simulink model "distributed_project_square"  (R2025b)
settings: Solver=VariableStepAuto  StartTime=0.0  StopTime=10  RelTol=1e-3  AbsTol=1e-3  EnableMultiTasking=on
model workspace (MAT data in the model file):
  t_now = 10
  v = 1
values from neighbouring files (symbols this model uses):
  m = 20    [FirstRegression.m]
  msg_init =     [distributed_project_adjusted.mat]
  N = min([length(e1), length(e2), length(e3), N_max])    [10_runs_result_for_odometer.m]    (also in cc.m = min(length(e1), length(e2)); distributed_project_adjusted.mat = 100; distributed_stats.m = min([length(e1),length(e2),length(e3)]); ten_runs_result_for_odometer.m)
  r = 0.05    [distributed_project.mat]    (also in distributed_project_adjusted.mat)
undefined symbols (not defined in the file or in its folder): fractalcoef, X, Y, Z
libraries: nesl_utility x69, sm_lib x50, simulink x20, matrix_library x20, mspfiltlib x4, sensorgpslib x4, mspsensorlib x4
(part 1 of 5)
settings Model: Creator=root  LastModifiedBy=root
settings SolverCC: AutoScaleAbsTol=off  AlgebraicLoopSolver=TrustRegion  MaxZcPerStep=1.0
settings DataIOCC: LimitDataPoints=on  MaxDataPoints=10000
settings OptimizationCC: ReuseModelBlockBuffer=off  LifeSpan=inf
settings DebuggingCC: UnconnectedInputMsg=warning  UnconnectedOutputMsg=warning  UnconnectedLineMsg=warning  AllowSymbolicDim=off  SubsystemReferenceDiagnosticForUnitTest=warning  SFUnexpectedBacktrackingDiag=warning  SFNoUnconditionalDefaultTransitionDiag=warning  SFExecutionAtInitializationDiag=none  UnderSpecifiedDimensionMsg=warning  ArithmeticOperatorsInVariantConditions=warning
settings ModelReferenceCC: EnableRefExpFcnMdlSchedulingChecks=on
settings SFSimCC: SimUseLocalCustomCode=off  CustomCodeUndefinedFunction=UseInterfaceOnly
settings RTWCC: RTWUseLocalCustomCode=off  GPUComputeCapability=3.5  DLArmComputeVersion=19.05
settings CodeAppCC: StateflowObjectComments=on
settings GRTTargetCC: TargetLangStandard=C89/C90 (ANSI)
settings ConfigComp: CovMetricSettings=dw  CovSaveCumulativeToWorkspaceVar=on  CovSaveSingleToWorkspaceVar=on  CovExternalEMLEnable=off  CovSFcnEnable=off
settings SimscapeCC: SimscapeLogType=all  SimscapeLogSimulationStatistics=on  SimscapeLogDataHistory=10000.0

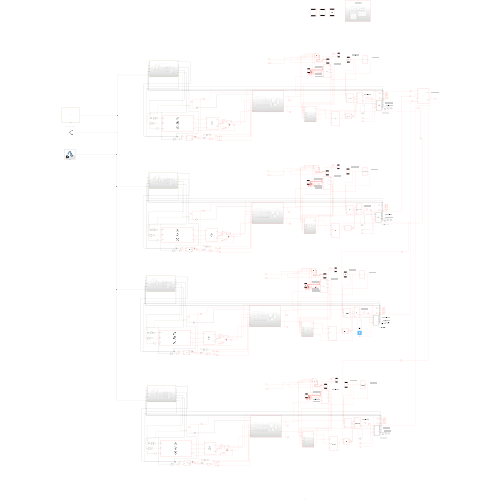
[thumbnail: Simulink's stored preview of the top-level diagram]
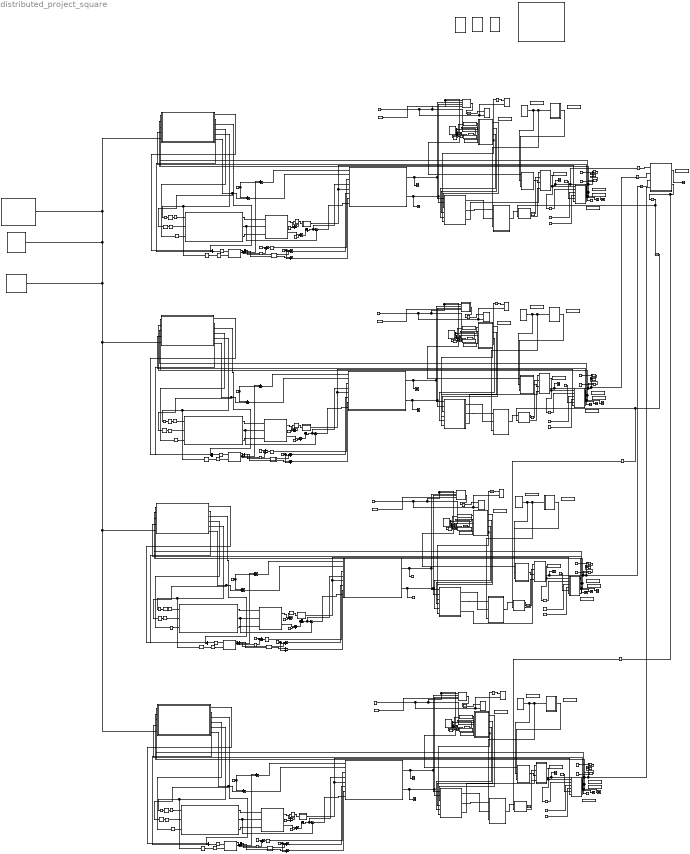
== system distributed_project_square ==
  AHRS{,1..3} (4 alike) : mspfiltlib/AHRS  DispRefFrame=NED  DecimationFactor=1  InitialProcessNoise=ahrsfilter.defaultProcessNoise  OrientationFormat=quaternion  SimulateUsing=Interpreted execution  AccelerometerNoise=0.0001924722  GyroscopeNoise=9.1385e-5  MagnetometerNoise=0.1  GyroscopeDriftNoise=3.0462e-13  LinearAccelerationNoise=0.0096236100000000012  MagneticDisturbanceNoise=0.5  LinearAccelerationDecayFactor=0.5  MagneticDisturbanceDecayFactor=0.5  ExpectedMagneticFieldStrength=50
  Add{1..28} (28 alike) : Sum
  Band-Limited White Noise{,1..19} (20 alike) : simulink/Sources/Band-Limited White Noise  Cov=[0.1]  Ts=0.01  seed=[23341]
  Bus Selector{,1..3} (4 alike) : BusSelector  OutputSignals=ID,x,P,t
  Constant : Constant  Value=2  OutDataTypeStr=int32  SampleTime=0.01
  Constant1 : Constant  OutDataTypeStr=int32  SampleTime=0.01
  Constant{4,7,10..11} (4 alike) : Constant  Value=0.8  SampleTime=0.01
  Constant2 : Constant  Value=3  OutDataTypeStr=int32  SampleTime=0.01
  Constant{3,6,8..9} (4 alike) : Constant  Value=0.0  SampleTime=0.01
  Constant5 : Constant  Value=4  OutDataTypeStr=int32  SampleTime=0.01
  Data Store Memory : DataStoreMemory  DataStoreName=msg_in  WriteAfterWriteMsg=warning  InitialValue=msg_init  ShowAdditionalParam=off  OutDataTypeStr=Bus: msgBus  Dimensions=MAX_AGENTS
  Data Store Memory1 : DataStoreMemory  DataStoreName=N  WriteAfterWriteMsg=warning  InitialValue=1  ShowAdditionalParam=off  OutDataTypeStr=double  Dimensions=MAX_AGENTS
  Data Store Memory2 : DataStoreMemory  DataStoreName=N_final  WriteAfterWriteMsg=warning  InitialValue=MAX_AGENTS  ShowAdditionalParam=off
  Data Store Read{,2,4,6} (4 alike) : DataStoreRead  DataStoreName=msg_in  SampleTime=0.01  DataStoreElements=msg_in  IndexOptions=Index vector (dialog)  Indices=1  OutputSizes=1
  Data Store Read{1,3,5,7} (4 alike) : DataStoreRead  DataStoreName=N_final  SampleTime=0.01  IndexOptions=Index vector (dialog)  Indices=1  OutputSizes=1
  Data Store Write{,2,4,6} (4 alike) : DataStoreWrite  DataStoreName=msg_in  SampleTime=0.01  DataStoreElements=msg_in  EnableIndexing=on  IndexOptions=Index vector (port)  Indices=1  OutputSizes=1
  Data Store Write{1,3,5,7} (4 alike) : DataStoreWrite  DataStoreName=N  SampleTime=0.01  EnableIndexing=on  IndexOptions=Index vector (port)  Indices=1  OutputSizes=1
  Demux{1..8} (8 alike) : Demux  Outputs=3
  Derivative{,1..11} (12 alike) : Derivative
  Digital Clock{,1..7} (8 alike) : DigitalClock  SampleTime=0.01
  Display{,1..40} (41 alike) : DisplayBlock  LabelPosition=Hide  Transparency=1  GridColor=[0.502, 0.502, 0.502]
  GPS{,1..3} (4 alike) : sensorgpslib/GPS  DispRefFrame=NED  PositionInputFormat=Local  ReferenceLocation=[ 0, 0, 0 ]  HorizontalPositionAccuracy=1.6  VerticalPositionAccuracy=3  VelocityAccuracy=0.1  DecayFactor=0.999  SeedDouble=67  SimulateUsing=Interpreted execution
      settings: LibrarySourceBlock=mspsensorlib/GPS
  IMU{,1..3} (4 alike) : mspsensorlib/IMU  DispRefFrame=NED  TemperaturePort=off  Temperature=25  MagneticFieldPort=off  MagneticFieldNED=[ 27.5550, -2.4169, -16.0849 ]  MagneticFieldENU=[ -2.4169, 27.5550, 16.0849 ]  SeedDouble=67  SimulateUsing=Interpreted execution  AccelParamsMeasurementRange=Inf  AccelParamsResolution=0  AccelParamsConstantBias=[ 0, 0, 0 ]  AccelParamsAxesMisalignment=[ 100, 0, 0; 0, 100, 0; 0, 0, 100 ]  AccelParamsNoiseDensity=[ 0, 0, 0 ]  AccelParamsBiasInstability=[ 0, 0, 0 ]  AccelParamsBiasInstabilityNumerator=fractalcoef().Numerator  AccelParamsBiasInstabilityDenominator=fractalcoef().Denominator  AccelParamsRandomWalk=[ 0, 0, 0 ]  AccelParamsNoiseType=double-sided  AccelParamsTemperatureBias=[ 0, 0, 0 ]  AccelParamsTemperatureScaleFactor=[ 0, 0, 0 ]  GyroParamsMeasurementRange=Inf  GyroParamsResolution=0  GyroParamsConstantBias=[ 0, 0, 0 ]  GyroParamsAxesMisalignment=[ 100, 0, 0; 0, 100, 0; 0, 0, 100 ]  GyroParamsAccelerationBias=[ 0, 0, 0 ]  GyroParamsNoiseDensity=[ 0, 0, 0 ]  GyroParamsBiasInstability=[ 0, 0, 0 ]  GyroParamsBiasInstabilityNumerator=fractalcoef().Numerator  GyroParamsBiasInstabilityDenominator=fractalcoef().Denominator  GyroParamsRandomWalk=[ 0, 0, 0 ]  GyroParamsNoiseType=double-sided  GyroParamsTemperatureBias=[ 0, 0, 0 ]  GyroParamsTemperatureScaleFactor=[ 0, 0, 0 ]  MagParamsMeasurementRange=Inf  MagParamsResolution=0  MagParamsConstantBias=[ 0, 0, 0 ]  MagParamsAxesMisalignment=[ 100, 0, 0; 0, 100, 0; 0, 0, 100 ]  MagParamsNoiseDensity=[ 0, 0, 0 ]  MagParamsBiasInstability=[ 0, 0, 0 ]  MagParamsBiasInstabilityNumerator=fractalcoef().Numerator  MagParamsBiasInstabilityDenominator=fractalcoef().Denominator  MagParamsRandomWalk=[ 0, 0, 0 ]  MagParamsNoiseType=double-sided  MagParamsTemperatureBias=[ 0, 0, 0 ]  MagParamsTemperatureScaleFactor=[ 0, 0, 0 ]
  L{,1..3} (4 alike) : Constant  Value=0.04  SampleTime=0.01
  Logical Operator{,1..3} (4 alike) : Logic  AllPortsSameDT=off  OutDataTypeStr=boolean
  MATLAB Function : MATLAB Function  TreatAsAtomicUnit=on
  MATLAB Function1 : MATLAB Function  TreatAsAtomicUnit=on
  MATLAB Function10 : MATLAB Function  TreatAsAtomicUnit=on
  MATLAB Function11 : MATLAB Function  TreatAsAtomicUnit=on
  MATLAB Function12 : MATLAB Function  TreatAsAtomicUnit=on
  MATLAB Function13 : MATLAB Function  TreatAsAtomicUnit=on
  MATLAB Function14 : MATLAB Function  TreatAsAtomicUnit=on
  MATLAB Function15 : MATLAB Function  TreatAsAtomicUnit=on
  MATLAB Function16 : MATLAB Function  TreatAsAtomicUnit=on
  MATLAB Function17 : MATLAB Function  TreatAsAtomicUnit=on
  MATLAB Function18 : MATLAB Function  TreatAsAtomicUnit=on
  MATLAB Function19 : MATLAB Function  TreatAsAtomicUnit=on
  MATLAB Function2 : MATLAB Function  TreatAsAtomicUnit=on
  MATLAB Function20 : MATLAB Function  TreatAsAtomicUnit=on
  MATLAB Function21 : MATLAB Function  TreatAsAtomicUnit=on
  MATLAB Function22 : MATLAB Function  TreatAsAtomicUnit=on
  MATLAB Function23 : MATLAB Function  TreatAsAtomicUnit=on
  MATLAB Function24 : MATLAB Function  TreatAsAtomicUnit=on
  MATLAB Function25 : MATLAB Function  TreatAsAtomicUnit=on
  MATLAB Function26 : MATLAB Function  TreatAsAtomicUnit=on
  MATLAB Function27 : MATLAB Function  TreatAsAtomicUnit=on
  MATLAB Function28 : MATLAB Function  TreatAsAtomicUnit=on
  MATLAB Function29 : MATLAB Function  TreatAsAtomicUnit=on
  MATLAB Function3 : MATLAB Function  TreatAsAtomicUnit=on
  MATLAB Function30 : MATLAB Function  TreatAsAtomicUnit=on
  MATLAB Function31 : MATLAB Function  TreatAsAtomicUnit=on
  MATLAB Function32 : MATLAB Function  TreatAsAtomicUnit=on
  MATLAB Function33 : MATLAB Function  TreatAsAtomicUnit=on
  MATLAB Function34 : MATLAB Function  TreatAsAtomicUnit=on
  MATLAB Function35 : MATLAB Function  TreatAsAtomicUnit=on
  MATLAB Function36 : MATLAB Function  TreatAsAtomicUnit=on
  MATLAB Function37 : MATLAB Function  TreatAsAtomicUnit=on
  MATLAB Function38 : MATLAB Function  TreatAsAtomicUnit=on
  MATLAB Function39 : MATLAB Function  TreatAsAtomicUnit=on
  MATLAB Function4 : MATLAB Function  TreatAsAtomicUnit=on
  MATLAB Function40 : MATLAB Function  TreatAsAtomicUnit=on
  MATLAB Function5 : MATLAB Function  TreatAsAtomicUnit=on
  MATLAB Function6 : MATLAB Function  TreatAsAtomicUnit=on
  MATLAB Function7 : MATLAB Function  TreatAsAtomicUnit=on
  MATLAB Function8 : MATLAB Function  TreatAsAtomicUnit=on
  MATLAB Function9 : MATLAB Function  TreatAsAtomicUnit=on
  Mechanism Configuration : sm_lib/Utilities/Mechanism Configuration  UniformGravity=Constant  GravityVector=[0 0 -9.80665]  GravityVectorUnits=m/s^2  LinearizationDelta=0.001  JointModeTransitionNonlinearIterations=2
  Rate Transition{,1..23} (24 alike) : RateTransition  OutPortSampleTime=0.01
  Relational Operator{,2,4,6} (4 alike) : RelationalOperator  OutDataTypeStr=boolean  ZeroCross=off  RndMeth=Simplest
  Relational Operator{1,3,5,7} (4 alike) : RelationalOperator  Operator=<  OutDataTypeStr=boolean  ZeroCross=off  RndMeth=Simplest
  Scope{,1..32} (33 alike) : Scope
      Scope settings: ActiveDisplayYMinimum=-1  ActiveDisplayYMaximum=1
      Scope1 settings: ActiveDisplayYMinimum=-0.0052486365636922527  ActiveDisplayYMaximum=0.047237729073230282
      Scope10 settings: ActiveDisplayYMinimum=-4.4781969660344139  ActiveDisplayYMaximum=2.0293339409947047  DataLoggingVariableName=ScopeData7
      Scope11 settings: ActiveDisplayYMinimum=-4.4781969660344139  ActiveDisplayYMaximum=2.0293339409947047  DataLoggingVariableName=ScopeData8
      Scope12 settings: ActiveDisplayYMinimum=-15.569158449616364  ActiveDisplayYMaximum=23.697536314281528  DataLoggingVariableName=ScopeData9
      Scope13 settings: ActiveDisplayYMinimum=-52.700432979002386  ActiveDisplayYMaximum=36.309061082783131  DataLoggingVariableName=ScopeData10
      Scope14 settings: ActiveDisplayYMinimum=-2292.39587890845  ActiveDisplayYMaximum=1608.5985281190563  DataLoggingVariableName=ScopeData11
      Scope15 settings: ActiveDisplayYMinimum=-1170.5511772576685  ActiveDisplayYMaximum=1424.4491042701625  DataLoggingVariableName=ScopeData12
      Scope16 settings: ActiveDisplayYMinimum=-1  ActiveDisplayYMaximum=1  DataLoggingVariableName=ScopeData16
      Scope17 settings: ActiveDisplayYMinimum=-0.0052486365636922527  ActiveDisplayYMaximum=0.047237729073230282  DataLoggingVariableName=ScopeData17
      Scope18 settings: ActiveDisplayYMinimum=-0.014006554084586675  ActiveDisplayYMaximum=0.057439431306869307  DataLoggingVariableName=ScopeData18
      Scope19 settings: ActiveDisplayYMinimum=-15.569158449616364  ActiveDisplayYMaximum=23.697536314281528  DataLoggingVariableName=ScopeData19
      Scope2 settings: ActiveDisplayYMinimum=-0.014006554084586675  ActiveDisplayYMaximum=0.057439431306869307  DataLoggingVariableName=ScopeData2
      Scope20 settings: ActiveDisplayYMinimum=-4.4781969660344139  ActiveDisplayYMaximum=2.0293339409947047  DataLoggingVariableName=ScopeData20
      Scope21 settings: ActiveDisplayYMinimum=-5.9275659718784439  ActiveDisplayYMaximum=7.4792876771773171  DataLoggingVariableName=ScopeData21
      Scope22 settings: ActiveDisplayYMinimum=-4.4781969660344139  ActiveDisplayYMaximum=2.0293339409947047  DataLoggingVariableName=ScopeData22
      Scope23 settings: ActiveDisplayYMinimum=-15.569158449616364  ActiveDisplayYMaximum=23.697536314281528  DataLoggingVariableName=ScopeData23
      Scope24 settings: ActiveDisplayYMinimum=-52.700432979002386  ActiveDisplayYMaximum=36.309061082783131  DataLoggingVariableName=ScopeData24
      Scope25 settings: ActiveDisplayYMinimum=-2292.39587890845  ActiveDisplayYMaximum=1608.5985281190563  DataLoggingVariableName=ScopeData25
      Scope26 settings: ActiveDisplayYMinimum=-1170.5511772576685  ActiveDisplayYMaximum=1424.4491042701625  DataLoggingVariableName=ScopeData26
      Scope27 settings: ActiveDisplayYMinimum=-52.700432979002386  ActiveDisplayYMaximum=36.309061082783131  DataLoggingVariableName=ScopeData27
      Scope28 settings: ActiveDisplayYMinimum=-2292.39587890845  ActiveDisplayYMaximum=1608.5985281190563  DataLoggingVariableName=ScopeData28
      Scope29 settings: ActiveDisplayYMinimum=-1170.5511772576685  ActiveDisplayYMaximum=1424.4491042701625  DataLoggingVariableName=ScopeData29
      Scope3 settings: ActiveDisplayYMinimum=-15.569158449616364  ActiveDisplayYMaximum=23.697536314281528  DataLoggingVariableName=ScopeData3
      Scope30 settings: ActiveDisplayYMinimum=-1  ActiveDisplayYMaximum=1  DataLoggingVariableName=ScopeData30
      Scope31 settings: ActiveDisplayYMinimum=-0.0052486365636922527  ActiveDisplayYMaximum=0.047237729073230282  DataLoggingVariableName=ScopeData31
      Scope32 settings: ActiveDisplayYMinimum=-0.014006554084586675  ActiveDisplayYMaximum=0.057439431306869307  DataLoggingVariableName=ScopeData32
      Scope4 settings: ActiveDisplayYMinimum=-52.700432979002386  ActiveDisplayYMaximum=36.309061082783131  DataLoggingVariableName=ScopeData4
      Scope5 settings: ActiveDisplayYMinimum=-2292.39587890845  ActiveDisplayYMaximum=1608.5985281190563  DataLoggingVariableName=ScopeData5
      Scope6 settings: ActiveDisplayYMinimum=-1170.5511772576685  ActiveDisplayYMaximum=1424.4491042701625  DataLoggingVariableName=ScopeData6
      Scope7 settings: ActiveDisplayYMinimum=-1  ActiveDisplayYMaximum=1  DataLoggingVariableName=ScopeData13
      Scope8 settings: ActiveDisplayYMinimum=-0.0052486365636922527  ActiveDisplayYMaximum=0.047237729073230282  DataLoggingVariableName=ScopeData14
      Scope9 settings: ActiveDisplayYMinimum=-0.014006554084586675  ActiveDisplayYMaximum=0.057439431306869307  DataLoggingVariableName=ScopeData15
  Selector{,1..3} (4 alike) : Selector  InputPortWidth=7  IndexOptions=Index vector (dialog)  Indices=1  OutputSizes=1
  Solver Configuration : nesl_utility/Solver Configuration  PhysicalDomain=network_engine_domain  SubClassName=solver  LeftPortType=input  RightPortType=generic  Tones=[]  Harmonics=[]  SimulateNoise=off  Profile=off  UseLocalSampling=off  EnableSwitchedLinearOptims=on  FrequencyDomain=off  UseCCode=off  RelTol=0.001  AbsTol=1e-06  MinStep=1e-09  ToWorkspace=off  RevertToSquareIcSolve=off  NumHomotopyIterations=100  PhasorMode=off  PhasorModeNumHarmonics=1  ConsistencySolver=NEWTON_XTOL_AFTER_FTOL  IndexReductionMethod=DerivativeReplacement  DoDC=off  ResidualTolerance=1e-09  ConsistencyTolSource=GLOBAL  ConsistencyAbsTol=0.001  ConsistencyRelTol=0.001  ConsistencyTolFactor=0.001  UseLocalSolver=off  LocalSolverChoice=NE_BACKWARD_EULER_ADVANCER  ResolveIndetEquations=on  FunctionEvalNumThread=1  LocalSolverSampleTime=0.001  DoFixedCost=off  MaxNonlinIter=3  MaxModeIter=2  ComputeImpulses=off  ImpulseIterations=2  LinearAlgebra=Sparse  LinearAlgebraNumThread=0  EquationFormulation=NE_TIME_EF  DelaysMemoryBudget=1024  AutomaticFiltering=on  FilteringTimeConstant=0.001  PartitionStorageMethod=AS_NEEDED  PartitionMemoryBudget=1024  PartitionMethod=FAST  MultibodyUseLocalSolver=off  MultibodyLocalSolverChoice=ODE2  MultibodyLocalSolverSampleTime=0.001
  Subsystem : Subsystem
  Subsystem1 : Subsystem
  Subsystem10 : Subsystem
  Subsystem11 : Subsystem
  Subsystem12 : Subsystem
  Subsystem2 : Subsystem
  Subsystem3 : Subsystem
  Subsystem4 : Subsystem
  Subsystem5 : Subsystem
  Subsystem6 : Subsystem
  Subsystem7 : Subsystem
  Subsystem8 : Subsystem
  Subsystem9 : Subsystem
  Subtract{,1..3} (4 alike) : Sum  Inputs=||+|-
  Transpose{,1..15} (16 alike) : matrix_library/Transpose
  Unit Delay{,2,13,16} (4 alike) : UnitDelay  InitialCondition=msg_init  SampleTime=0.01  HasFrameUpgradeWarning=on
  Unit Delay{1,3..12,14,17,19..20} (15 alike) : UnitDelay  SampleTime=0.01  HasFrameUpgradeWarning=on
  Vector Concatenate{,1..3} (4 alike) : Concatenate  NumInputs=3  Mode=Multidimensional array  ConcatenateDimension=2
  World Frame : sm_lib/Frames and Transforms/World Frame
  kd{,1..3} (4 alike) : Constant  Value=2.0  SampleTime=0.01
  kp : Constant  Value=1.5  SampleTime=0.01
  kp1 : Constant  Value=0.2  SampleTime=0.01
  kp2 : Constant  Value=1.0  SampleTime=0.01
  kp3 : Constant  Value=1.5  SampleTime=0.01
  wires:
  Derivative1/1 -> Transpose1/1
  Band-Limited White Noise/1 -> Add1/2, Add5/1
  IMU/1 -> AHRS/1
  IMU/2 -> Subtract/2, AHRS/2
  IMU/3 -> AHRS/3
  Subsystem1/1(x) -> Vector Concatenate/1
  Subsystem1/2(y) -> Vector Concatenate/2
  Subsystem1/3(z) -> Vector Concatenate/3
  Vector Concatenate/1 -> Rate Transition3/1
  Transpose/1 -> Rate Transition4/1
  Transpose1/1 -> Rate Transition2/1
  Subsystem1/6(w) -> Add5/2, Transpose2/1
  Add5/1 -> Subsystem/2(w_enc)
  Transpose2/1 -> Rate Transition1/1
  Subsystem1/4(q) -> Rate Transition/1
  Rate Transition/1 -> IMU/3
  Rate Transition1/1 -> IMU/2
  Rate Transition2/1 -> IMU/1
  Rate Transition3/1 -> GPS/1
  Rate Transition4/1 -> GPS/2
  AHRS/1 -> Add6/1
  GPS/1 -> Demux1/1
  Demux1/2 -> MATLAB Function/2(lon)
  Demux1/1 -> MATLAB Function/1(lat)
  AHRS/2 -> Add7/1
  MATLAB Function/1(x) -> Add9/1
  MATLAB Function/2(y) -> Add8/1
  Subsystem/1(x_hat) -> Scope3/1, Subsystem7/1(x_i_hat), MATLAB Function16/2(x_i)
  Subsystem/2(P_hat) -> Scope2/1, Subsystem7/2(P_i), MATLAB Function16/3(P_i)
  Constant1/1 -> Data Store Write1/2, Data Store Write/2, MATLAB Function16/1(ID_i), MATLAB Function4/1(ID_i), MATLAB Function2/2(my_id)
  Digital Clock/1 -> MATLAB Function16/4(t_now)
  Data Store Read/1 -> Selector/1, MATLAB Function2/1(msg_in)
  MATLAB Function2/1(x_hat_neighbors) -> Subsystem7/3(x_hat_neighbors)
  MATLAB Function2/2(neighbor_idx) -> Subsystem7/4(Neighbor_idx)
  Subsystem7/2(x_i_cons) -> MATLAB Function3/1(x_i_cons)
  MATLAB Function2/4(N) -> Subsystem7/6(N), Unit Delay1/1
  MATLAB Function3/1(x_c) -> MATLAB Function28/1("x_c_raw ")
  MATLAB Function4/1(delta_i) -> MATLAB Function6/3(delta_i)
  Derivative/1 -> MATLAB Function7/2(ei_vel)
  kp/1 -> MATLAB Function7/3(kp)
  kd/1 -> MATLAB Function7/4(kd)
  L/1 -> MATLAB Function7/5(L)
  Add1/1 -> Subsystem/1(v_enc)
  Band-Limited White Noise4/1 -> Add6/2
  Add6/1 -> Transpose4/1
  Band-Limited White Noise5/1 -> Add7/2
  Add7/1 -> Demux4/1
  Band-Limited White Noise6/1 -> Add8/2, Add9/2
  Add8/1 -> Subsystem/7(gps_y)
  Add9/1 -> Subsystem/6(gps_x)
  Subtract/1 -> Subsystem/8(gyro_bias)
  MATLAB Function2/3(P_j_neighbours) -> Subsystem7/5(P_j_neighbors)
  Subsystem7/1(Neighbours) -> MATLAB Function3/2(x_hat_neighbors)
  MATLAB Function5/1(formation) -> MATLAB Function4/3(formation)
  Data Store Read1/1 -> MATLAB Function4/2(N), MATLAB Function3/3(N_all), MATLAB Function5/1(N_final)
  Unit Delay1/1 -> Data Store Write1/1
  Demux4/3 -> Subsystem/4(w_imu), Subtract/1
  MATLAB Function16/1(msg) -> Unit Delay/1
  Unit Delay/1 -> Data Store Write/1
  MATLAB Function7/1(vL) -> Scope5/1, Subsystem1/1(vL)
  MATLAB Function7/2(vR) -> Scope6/1, Subsystem1/2(vR)
  Subsystem1/5(v) -> Transpose/1, Derivative1/1
  Digital Clock5/1 -> MATLAB Function2/3(t_now)
  Bus Selector/2 -> Scope/1  "<x>"
  Bus Selector/3 -> Scope1/1  "<P>"
  Bus Selector/1 -> ?  "<ID>"
  Bus Selector/4 -> ?  "<t>"
  Selector/1 -> Bus Selector/1
  Transpose4/1 -> MATLAB Function24/1(quat)
  MATLAB Function24/1(theta) -> MATLAB Function7/6(theta), Subsystem/5(theta_imu)
  GPS/2 -> Derivative5/1, Add1/1
  Add10/1 -> Rate Transition15/1
  Band-Limited White Noise7/1 -> Add10/2
  Rate Transition15/1 -> Subsystem/3(a)
  Derivative5/1 -> Add10/1
  MATLAB Function7/3(w_scaled) -> Scope4/1, Subsystem1/3(w_scaled)
  Constant3/1 -> Relational Operator/2
  Constant4/1 -> Relational Operator1/2
  Relational Operator/1 -> Logical Operator/1
  Relational Operator1/1 -> Logical Operator/2
  MATLAB Function6/1(ei_pos_f) -> MATLAB Function7/1(ei_pos), Derivative/1
  MATLAB Function6/2(ei_norm) -> Scope22/1, Unit Delay7/1, Relational Operator1/1, Relational Operator/1
  MATLAB Function7/4(u) -> Subsystem1/4(u)
  MATLAB Function27/1(formation_achieved) -> Scope21/1
  Subsystem7/3(x_fused) -> MATLAB Function6/1(x_fused)
  MATLAB Function28/1(x_c_out) -> Unit Delay6/1
  Unit Delay7/1 -> MATLAB Function27/1(ei_norm_1)
  Unit Delay8/1 -> MATLAB Function27/2(ei_norm_2)
  Unit Delay9/1 -> MATLAB Function27/3(ei_norm_3)
  Subsystem4/1(x) -> Vector Concatenate1/1
  MATLAB Function18/2(vR) -> Scope15/1, Subsystem4/2(vR)
  Bus Selector1/2 -> Scope7/1  "<x>"
  MATLAB Function9/3(P_j_neighbours) -> Subsystem5/5(P_j_neighbors)
  Demux3/3 -> Subsystem3/4(w_imu), Subtract1/1
  IMU1/1 -> AHRS1/1
  Subsystem5/1(Neighbours) -> MATLAB Function13/2(x_hat_neighbors)
  Subsystem4/2(y) -> Vector Concatenate1/2
  Derivative2/1 -> MATLAB Function18/2(ei_vel)
  Subsystem5/3(x_fused) -> MATLAB Function17/1(x_fused)
  Selector1/1 -> Bus Selector1/1
  MATLAB Function9/4(N) -> Subsystem5/6(N), Unit Delay3/1
  Vector Concatenate1/1 -> Rate Transition9/1
  L1/1 -> MATLAB Function18/5(L)
  Subsystem4/4(q) -> Rate Transition5/1
  Unit Delay2/1 -> Data Store Write2/1
  IMU1/3 -> AHRS1/3
  Data Store Read3/1 -> MATLAB Function14/2(N), MATLAB Function13/3(N_all), MATLAB Function15/1(N_final)
  Derivative3/1 -> Transpose5/1
  MATLAB Function18/4(u) -> Subsystem4/4(u)
  MATLAB Function1/1(x) -> Add14/1
  Subtract1/1 -> Subsystem3/8(gyro_bias)
  MATLAB Function9/1(x_hat_neighbors) -> Subsystem5/3(x_hat_neighbors)
  Add12/1 -> Demux3/1
  MATLAB Function10/1(theta) -> MATLAB Function18/6(theta), Subsystem3/5(theta_imu)
  Subsystem3/2(P_hat) -> Scope9/1, Subsystem5/2(P_i), MATLAB Function8/3(P_i)
  Digital Clock1/1 -> MATLAB Function8/4(t_now)
  Transpose5/1 -> Rate Transition8/1
  Demux2/2 -> MATLAB Function1/2(lon)
  Transpose6/1 -> Rate Transition6/1
  MATLAB Function1/2(y) -> Add13/1
  AHRS1/2 -> Add12/1
  MATLAB Function18/1(vL) -> Scope14/1, Subsystem4/1(vL)
  Digital Clock2/1 -> MATLAB Function9/3(t_now)
  Rate Transition7/1 -> Subsystem3/3(a)
  MATLAB Function13/1(x_c) -> MATLAB Function12/1("x_c_raw ")
  Relational Operator2/1 -> Logical Operator1/1
  Band-Limited White Noise1/1 -> Add2/2, Add4/1
  MATLAB Function17/2(ei_norm) -> Scope11/1, Relational Operator3/1, Unit Delay8/1, Relational Operator2/1
  Add14/1 -> Subsystem3/6(gps_x)
  GPS1/1 -> Demux2/1
  Add3/1 -> Rate Transition7/1
  Constant7/1 -> Relational Operator3/2
  GPS1/2 -> Derivative4/1, Add2/1
  Transpose7/1 -> MATLAB Function10/1(quat)
  Derivative4/1 -> Add3/1
  Rate Transition10/1 -> GPS1/2
  Subsystem3/1(x_hat) -> Scope12/1, Subsystem5/1(x_i_hat), MATLAB Function8/2(x_i)
  Subsystem5/2(x_i_cons) -> MATLAB Function13/1(x_i_cons)
  Bus Selector1/3 -> Scope8/1  "<P>"
  Data Store Read2/1 -> Selector1/1, MATLAB Function9/1(msg_in)
  Add4/1 -> Subsystem3/2(w_enc)
  Subsystem4/6(w) -> Add4/2, Transpose6/1
  MATLAB Function9/2(neighbor_idx) -> Subsystem5/4(Neighbor_idx)
  Subsystem4/5(v) -> Transpose3/1, Derivative3/1
  Band-Limited White Noise2/1 -> Add11/2
  Demux2/1 -> MATLAB Function1/1(lat)
  MATLAB Function18/3(w_scaled) -> Scope13/1, Subsystem4/3(w_scaled)
  MATLAB Function15/1(formation) -> MATLAB Function14/3(formation)
  Add2/1 -> Subsystem3/1(v_enc)
  kp1/1 -> MATLAB Function18/3(kp)
  Subsystem4/3(z) -> Vector Concatenate1/3
  Rate Transition5/1 -> IMU1/3
  MATLAB Function8/1(msg) -> Unit Delay2/1
  Relational Operator3/1 -> Logical Operator1/2
  IMU1/2 -> Subtract1/2, AHRS1/2
  Rate Transition9/1 -> GPS1/1
  kd1/1 -> MATLAB Function18/4(kd)
  Band-Limited White Noise3/1 -> Add12/2
  AHRS1/1 -> Add11/1
  Add13/1 -> Subsystem3/7(gps_y)
  Rate Transition6/1 -> IMU1/2
  Constant/1 -> MATLAB Function8/1(ID_i), MATLAB Function14/1(ID_i), MATLAB Function9/2(my_id), Data Store Write3/2, Data Store Write2/2
  MATLAB Function12/1(x_c_out) -> Unit Delay12/1
  Constant6/1 -> Relational Operator2/2
  MATLAB Function17/1(ei_pos_f) -> MATLAB Function18/1(ei_pos), Derivative2/1
  Band-Limited White Noise8/1 -> Add13/2, Add14/2
  Unit Delay3/1 -> Data Store Write3/1
  Transpose3/1 -> Rate Transition10/1
  Band-Limited White Noise9/1 -> Add3/2
  Rate Transition8/1 -> IMU1/1
  Add11/1 -> Transpose7/1
  MATLAB Function14/1(delta_i) -> MATLAB Function17/3(delta_i)
  Bus Selector1/1 -> ?  "<ID>"
  Bus Selector1/4 -> ?  "<t>"
  Subsystem8/1(x) -> Vector Concatenate2/1
  MATLAB Function32/2(vR) -> Scope26/1, Subsystem8/2(vR)
  Bus Selector2/2 -> Scope16/1  "<x>"
  MATLAB Function21/3(P_j_neighbours) -> Subsystem9/5(P_j_neighbors)
  Demux6/3 -> Subsystem6/4(w_imu), Subtract2/1
  IMU2/1 -> AHRS2/1
  Subsystem9/1(Neighbours) -> MATLAB Function26/2(x_hat_neighbors)
  Subsystem8/2(y) -> Vector Concatenate2/2
  Derivative6/1 -> MATLAB Function32/2(ei_vel)
  Subsystem9/3(x_fused) -> MATLAB Function31/1(x_fused)
  Selector2/1 -> Bus Selector2/1
  MATLAB Function21/4(N) -> Subsystem9/6(N), Unit Delay17/1
  Vector Concatenate2/1 -> Rate Transition16/1
  L2/1 -> MATLAB Function32/5(L)
  Subsystem8/4(q) -> Rate Transition11/1
  Unit Delay16/1 -> Data Store Write4/1
  IMU2/3 -> AHRS2/3
  Data Store Read5/1 -> MATLAB Function29/2(N), MATLAB Function26/3(N_all), MATLAB Function30/1(N_final)
  Derivative7/1 -> Transpose9/1
  MATLAB Function32/4(u) -> Subsystem8/4(u)
  MATLAB Function19/1(x) -> Add21/1
  Subtract2/1 -> Subsystem6/8(gyro_bias)
  MATLAB Function21/1(x_hat_neighbors) -> Subsystem9/3(x_hat_neighbors)
  Add19/1 -> Demux6/1
  MATLAB Function22/1(theta) -> MATLAB Function32/6(theta), Subsystem6/5(theta_imu)
  Subsystem6/2(P_hat) -> Scope18/1, Subsystem9/2(P_i), MATLAB Function20/3(P_i)
  Digital Clock3/1 -> MATLAB Function20/4(t_now)
  Transpose9/1 -> Rate Transition14/1
  Demux5/2 -> MATLAB Function19/2(lon)
  Transpose10/1 -> Rate Transition12/1
  MATLAB Function19/2(y) -> Add20/1
  AHRS2/2 -> Add19/1
  MATLAB Function32/1(vL) -> Scope25/1, Subsystem8/1(vL)
  Digital Clock4/1 -> MATLAB Function21/3(t_now)
  Rate Transition13/1 -> Subsystem6/3(a)
  MATLAB Function26/1(x_c) -> MATLAB Function25/1("x_c_raw ")
  Relational Operator4/1 -> Logical Operator2/1
  Band-Limited White Noise10/1 -> Add15/2, Add17/1
  MATLAB Function31/2(ei_norm) -> Scope20/1, Relational Operator5/1, Unit Delay9/1, Relational Operator4/1
  Add21/1 -> Subsystem6/6(gps_x)
  GPS2/1 -> Demux5/1
  Add16/1 -> Rate Transition13/1
  Constant10/1 -> Relational Operator5/2
  GPS2/2 -> Derivative8/1, Add15/1
  Transpose11/1 -> MATLAB Function22/1(quat)
  Derivative8/1 -> Add16/1
  Rate Transition17/1 -> GPS2/2
  Subsystem6/1(x_hat) -> Scope23/1, Subsystem9/1(x_i_hat), MATLAB Function20/2(x_i)
  Subsystem9/2(x_i_cons) -> MATLAB Function26/1(x_i_cons)
  Bus Selector2/3 -> Scope17/1  "<P>"
  Data Store Read4/1 -> Selector2/1, MATLAB Function21/1(msg_in)
  Add17/1 -> Subsystem6/2(w_enc)
  Subsystem8/6(w) -> Add17/2, Transpose10/1
  MATLAB Function21/2(neighbor_idx) -> Subsystem9/4(Neighbor_idx)
  Subsystem8/5(v) -> Transpose8/1, Derivative7/1
  Band-Limited White Noise11/1 -> Add18/2
  Demux5/1 -> MATLAB Function19/1(lat)
  MATLAB Function32/3(w_scaled) -> Scope24/1, Subsystem8/3(w_scaled)
  MATLAB Function30/1(formation) -> MATLAB Function29/3(formation)
  Add15/1 -> Subsystem6/1(v_enc)
  kp2/1 -> MATLAB Function32/3(kp)
  Subsystem8/3(z) -> Vector Concatenate2/3
  Rate Transition11/1 -> IMU2/3
  MATLAB Function20/1(msg) -> Unit Delay16/1
  Relational Operator5/1 -> Logical Operator2/2
  IMU2/2 -> Subtract2/2, AHRS2/2
  Rate Transition16/1 -> GPS2/1
  kd2/1 -> MATLAB Function32/4(kd)
  Band-Limited White Noise12/1 -> Add19/2
  AHRS2/1 -> Add18/1
  Add20/1 -> Subsystem6/7(gps_y)
  Rate Transition12/1 -> IMU2/2
  Constant2/1 -> MATLAB Function20/1(ID_i), MATLAB Function29/1(ID_i), MATLAB Function21/2(my_id), Data Store Write5/2, Data Store Write4/2
  MATLAB Function25/1(x_c_out) -> Unit Delay20/1
  Constant9/1 -> Relational Operator4/2
  MATLAB Function31/1(ei_pos_f) -> MATLAB Function32/1(ei_pos), Derivative6/1
  Band-Limited White Noise13/1 -> Add20/2, Add21/2
  Unit Delay17/1 -> Data Store Write5/1
  Transpose8/1 -> Rate Transition17/1
  Band-Limited White Noise14/1 -> Add16/2
  Rate Transition14/1 -> IMU2/1
  Add18/1 -> Transpose11/1
  MATLAB Function29/1(delta_i) -> MATLAB Function31/3(delta_i)
  Bus Selector2/1 -> ?  "<ID>"
  Bus Selector2/4 -> ?  "<t>"
  Unit Delay11/1 -> Unit Delay5/1, MATLAB Function12/2(all_converged)
  Unit Delay5/1 -> MATLAB Function25/2(all_converged)
  MATLAB Function27/2(all_converged) -> Unit Delay19/1, Unit Delay10/1
  Unit Delay10/1 -> MATLAB Function28/2(all_converged), Unit Delay11/1
  Unit Delay6/1 -> MATLAB Function6/2(x_c)
  Unit Delay12/1 -> MATLAB Function17/2(x_c)
  Unit Delay20/1 -> MATLAB Function31/2(x_c)
  MATLAB Function28/2(x_c_raw) -> MATLAB Function6/4(x_c_raw)
  MATLAB Function25/2(x_c_raw) -> MATLAB Function31/4(x_c_raw)
  MATLAB Function12/2(x_c_raw) -> MATLAB Function17/4(x_c_raw)
  ? -> ?
  Data Store Read7/1 -> MATLAB Function35/2(N), MATLAB Function34/3(N_all), MATLAB Function36/1(N_final)
  Constant8/1 -> Relational Operator6/2
  kp3/1 -> MATLAB Function38/3(kp)
  MATLAB Function40/1(x_hat_neighbors) -> Subsystem12/3(x_hat_neighbors)
  IMU3/2 -> Subtract3/2, AHRS3/2
  GPS3/1 -> Demux7/1
  AHRS3/1 -> Add22/1
  Unit Delay4/1 -> MATLAB Function37/2(x_c)
  IMU3/1 -> AHRS3/1
  MATLAB Function11/1(x) -> Add25/1
  Band-Limited White Noise17/1 -> Add23/2
  Band-Limited White Noise15/1 -> Add26/2, Add28/1
  MATLAB Function37/2(ei_norm) -> Scope10/1, Relational Operator7/1, MATLAB Function27/4(ei_norm_4), Relational Operator6/1
  Band-Limited White Noise19/1 -> Add27/2
  Rate Transition23/1 -> GPS3/1
  MATLAB Function40/4(N) -> Subsystem12/6(N), Unit Delay14/1
  Subsystem12/1(Neighbours) -> MATLAB Function34/2(x_hat_neighbors)
  Digital Clock7/1 -> MATLAB Function40/3(t_now)
  Rate Transition21/1 -> Subsystem10/3(a)
  GPS3/2 -> Derivative11/1, Add26/1
  Subsystem12/3(x_fused) -> MATLAB Function37/1(x_fused)
  MATLAB Function33/2(x_c_raw) -> MATLAB Function37/4(x_c_raw)
  Data Store Read6/1 -> Selector3/1, MATLAB Function40/1(msg_in)
  MATLAB Function33/1(x_c_out) -> Unit Delay4/1
  Derivative9/1 -> MATLAB Function38/2(ei_vel)
  Demux7/2 -> MATLAB Function11/2(lon)
  Transpose12/1 -> Rate Transition18/1
  Rate Transition22/1 -> IMU3/1
  Add23/1 -> Demux8/1
  MATLAB Function38/4(u) -> Subsystem11/4(u)
  Relational Operator6/1 -> Logical Operator3/1
  MATLAB Function40/3(P_j_neighbours) -> Subsystem12/5(P_j_neighbors)
  Bus Selector3/4 -> ?  "<t>"
  Transpose13/1 -> Rate Transition22/1
  Subsystem10/2(P_hat) -> Scope32/1, Subsystem12/2(P_i), MATLAB Function39/3(P_i)
  Add25/1 -> Subsystem10/6(gps_x)
  Selector3/1 -> Bus Selector3/1
  MATLAB Function39/1(msg) -> Unit Delay13/1
  Unit Delay13/1 -> Data Store Write6/1
  Subsystem11/6(w) -> Add28/2, Transpose14/1
  Subsystem11/1(x) -> Vector Concatenate3/1
  Digital Clock6/1 -> MATLAB Function39/4(t_now)
  Unit Delay14/1 -> Data Store Write7/1
  Band-Limited White Noise18/1 -> Add24/2, Add25/2
  Subsystem11/3(z) -> Vector Concatenate3/3
  Rate Transition20/1 -> IMU3/2
  Demux8/3 -> Subsystem10/4(w_imu), Subtract3/1
  MATLAB Function37/1(ei_pos_f) -> MATLAB Function38/1(ei_pos), Derivative9/1
  Subsystem11/5(v) -> Transpose12/1, Derivative10/1
  Demux7/1 -> MATLAB Function11/1(lat)
  Band-Limited White Noise16/1 -> Add22/2
  MATLAB Function40/2(neighbor_idx) -> Subsystem12/4(Neighbor_idx)
  Derivative10/1 -> Transpose13/1
  Rate Transition18/1 -> GPS3/2
  MATLAB Function38/1(vL) -> Scope28/1, Subsystem11/1(vL)
  L3/1 -> MATLAB Function38/5(L)
  Bus Selector3/2 -> Scope30/1  "<x>"
  MATLAB Function34/1(x_c) -> MATLAB Function33/1("x_c_raw ")
  AHRS3/2 -> Add23/1
  Subsystem10/1(x_hat) -> Scope19/1, Subsystem12/1(x_i_hat), MATLAB Function39/2(x_i)
  Add22/1 -> Transpose15/1
  Add28/1 -> Subsystem10/2(w_enc)
  Constant5/1 -> MATLAB Function39/1(ID_i), MATLAB Function35/1(ID_i), MATLAB Function40/2(my_id), Data Store Write7/2, Data Store Write6/2
  kd3/1 -> MATLAB Function38/4(kd)
  IMU3/3 -> AHRS3/3
  MATLAB Function23/1(theta) -> MATLAB Function38/6(theta), Subsystem10/5(theta_imu)
  Add27/1 -> Rate Transition21/1
  Vector Concatenate3/1 -> Rate Transition23/1
  Subsystem12/2(x_i_cons) -> MATLAB Function34/1(x_i_cons)
  Transpose14/1 -> Rate Transition20/1
  MATLAB Function35/1(delta_i) -> MATLAB Function37/3(delta_i)
  Bus Selector3/1 -> ?  "<ID>"
  MATLAB Function38/3(w_scaled) -> Scope27/1, Subsystem11/3(w_scaled)
  MATLAB Function38/2(vR) -> Scope29/1, Subsystem11/2(vR)
  Subsystem11/4(q) -> Rate Transition19/1
  Derivative11/1 -> Add27/1
  Add26/1 -> Subsystem10/1(v_enc)
  Bus Selector3/3 -> Scope31/1  "<P>"
  MATLAB Function11/2(y) -> Add24/1
  Rate Transition19/1 -> IMU3/3
  MATLAB Function36/1(formation) -> MATLAB Function35/3(formation)
  Add24/1 -> Subsystem10/7(gps_y)
  Transpose15/1 -> MATLAB Function23/1(quat)
  Relational Operator7/1 -> Logical Operator3/2
  Subtract3/1 -> Subsystem10/8(gyro_bias)
  Constant11/1 -> Relational Operator7/2
  Subsystem11/2(y) -> Vector Concatenate3/2
  Unit Delay19/1 -> MATLAB Function33/2(all_converged)
  connections:
  Mechanism Configuration/RConn1 -- Subsystem11/LConn1 -- Subsystem8/LConn1 -- Subsystem4/LConn1 -- Solver Configuration/RConn1 -- Subsystem1/LConn1 -- World Frame/RConn1

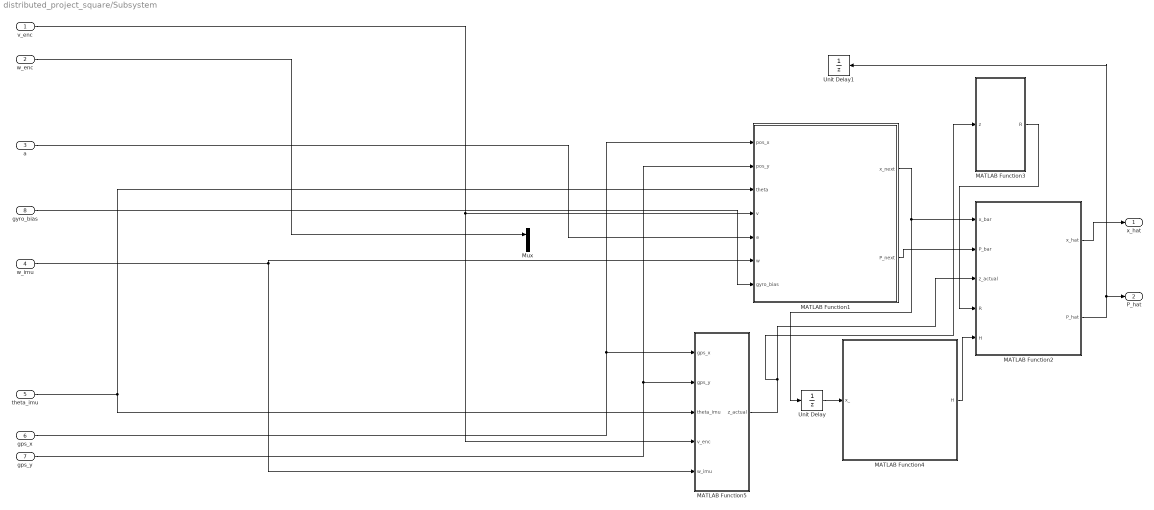
== system distributed_project_square/Subsystem ==
  v_enc : Inport  PortDimensions=[1 3]
  w_enc : Inport  Port=2
  a : Inport  Port=3
  w_imu : Inport  Port=4  PortDimensions=1
  theta_imu : Inport  Port=5
  gps_x : Inport  Port=6
  gps_y : Inport  Port=7
  gyro_bias : Inport  Port=8
  MATLAB Function1 : MATLAB Function  TreatAsAtomicUnit=on
  MATLAB Function2 : MATLAB Function  TreatAsAtomicUnit=on
  MATLAB Function3 : MATLAB Function  TreatAsAtomicUnit=on
  MATLAB Function4 : MATLAB Function  TreatAsAtomicUnit=on
  MATLAB Function5 : MATLAB Function  TreatAsAtomicUnit=on
  Mux : Mux  Inputs=2
  Unit Delay : UnitDelay  SampleTime=0.01  HasFrameUpgradeWarning=on
  Unit Delay1 : UnitDelay  SampleTime=0.01  HasFrameUpgradeWarning=on
  x_hat : Outport
  P_hat : Outport  Port=2
  wires:
  MATLAB Function2/2(P_hat) -> P_hat/1, Unit Delay1/1
  gps_y/1 -> MATLAB Function1/2(pos_y), MATLAB Function5/2(gps_y)
  theta_imu/1 -> MATLAB Function1/3(theta), MATLAB Function5/3(theta_imu)
  MATLAB Function5/1(z_actual) -> MATLAB Function3/1(z), MATLAB Function2/3(z_actual)
  MATLAB Function2/1(x_hat) -> x_hat/1
  MATLAB Function1/2(P_next) -> MATLAB Function2/2(P_bar)
  MATLAB Function4/1(H) -> MATLAB Function2/5(H)
  v_enc/1 -> MATLAB Function5/4(v_enc), MATLAB Function1/4(v)
  a/1 -> MATLAB Function1/5(a)
  gps_x/1 -> MATLAB Function1/1(pos_x), MATLAB Function5/1(gps_x)
  MATLAB Function1/1(x_next) -> Unit Delay/1, MATLAB Function2/1(x_bar)
  MATLAB Function3/1(R) -> MATLAB Function2/4(R)
  w_enc/1 -> Mux/1
  gyro_bias/1 -> MATLAB Function1/7(gyro_bias)
  Unit Delay/1 -> MATLAB Function4/1(x_)
  w_imu/1 -> MATLAB Function5/5(w_imu), MATLAB Function1/6(w)
